simulink model "gm_sampleModel1687_3_sub"  (R2023a)
settings: Solver=VariableStepAuto  StartTime=0.0  StopTime=10.0  RelTol=1e-3
libraries: hdlsllib x3, simulink x2
settings Model: Creator=user1  LastModifiedBy=user1
settings OptimizationCC: BlockReduction=off  ConditionallyExecuteInputs=off
settings DebuggingCC: InheritedTsInSrcMsg=none

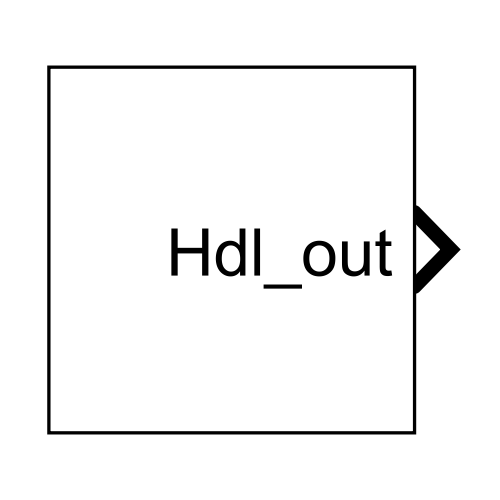
[thumbnail: Simulink's stored preview of the top-level diagram]
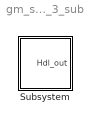
== system gm_sampleModel1687_3_sub ==
  Subsystem : Subsystem

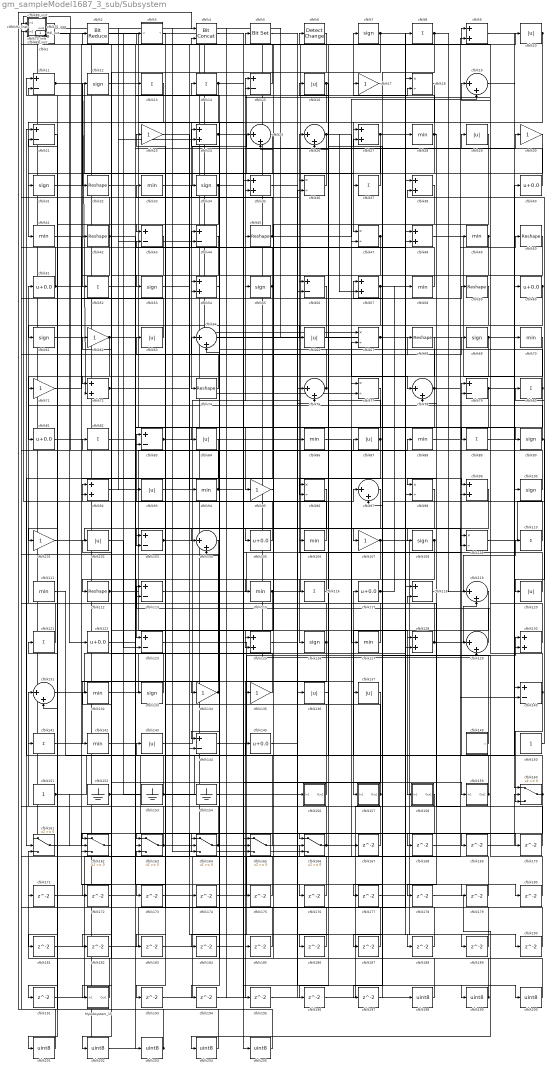
== system gm_sampleModel1687_3_sub/Subsystem ==
  Mysubsystem_15 : Subsystem
  cfblk1 : hdlsllib/Logic and Bit Operations/Bit Slice  lidx=7  ridx=0
  cfblk{10,16,29,63,66,84,87,93,102,120,136..137,143} (13 alike) : Abs  OutDataTypeStr=uint8  SaturateOnIntegerOverflow=off
  cfblk{7,12,31,34,53,55,61,69,90,100,108,126,133} (13 alike) : Signum
  cfblk{17,23,30,62,71,95,101,107,134..135} (10 alike) : Gain  OutDataTypeStr=uint8
  cfblk{11,15,21,43..44,56,79,83,103,113,118,123,140,144} (14 alike) : Sum  Inputs=+-  OutDataTypeStr=uint8
  cfblk{19,25..26,64,76,78,97,104,119,129,131} (11 alike) : Sum  Inputs=|++  OutDataTypeStr=uint8
  cfblk{40,51,60,81,105,117,122,145} (8 alike) : Bias  Bias=0.0  SaturateOnIntegerOverflow=off
  cfblk{28,33,41,49,58,70,86,88,94,106,111,115,127,132,142} (15 alike) : MinMax  OutDataTypeStr=uint8
  cfblk{18,36,47,67,77,96,98,109} (8 alike) : Product  Inputs=*/  OutDataTypeStr=uint8  RndMeth=Zero  SaturateOnIntegerOverflow=on
  cfblk{8,13..14,37,52,80,82,89,110,116,121,141} (12 alike) : Sum  Inputs=+  OutDataTypeStr=uint8
  cfblk{32,42,45,50,59,68,74,112} (8 alike) : Reshape
  cfblk114_inst : Subsystem
  cfblk124_inst : Subsystem
  cfblk{9,24,27,35,38,48,54,57,72,92,99,125,128,130} (14 alike) : Sum  OutDataTypeStr=uint8
  cfblk138_inst : Subsystem
  cfblk149 : Subsystem  mask(Counter Limited){uplimit=double(7), tsamp=double(-1)}
      mask prompts: uplimit "Simulink:masks:UpperLimit_MP"; tsamp "Simulink:masks:SampleTime_MP"
      mask help: Simulink:masks:CounterLimited_MD
      mask init:
      | nbits = double(8);
      | tsamp = double(-1);
      | uplimit = double(7);
  cfblk150 : Constant  OutDataTypeStr=uint8  SampleTime=-1
  cfblk151 : Constant  OutDataTypeStr=uint8  SampleTime=-1
  cfblk152 : Ground
  cfblk153 : Ground
  cfblk154 : Ground
  cfblk156 : Subsystem
  cfblk157 : Subsystem
  cfblk158 : Subsystem
  cfblk159 : Subsystem
  cfblk{160..166} (7 alike) : Switch  OutDataTypeStr=uint8  SaturateOnIntegerOverflow=off  InputSameDT=off
  cfblk{167..191,193..197} (30 alike) : Delay  SampleTime=1
  cfblk{198..205} (8 alike) : DataTypeConversion  OutDataTypeStr=uint8  SaturateOnIntegerOverflow=off  RndMeth=Floor
  cfblk2 : hdlsllib/Logic and Bit Operations/Bit Reduce  mode=AND
  cfblk20_inst : Subsystem
  cfblk22_inst : Subsystem
  cfblk3 : Subsystem  mask(Detect Rise Positive){vinit=double(0), InputProcessing=Elements as channels (sample based), OutDataTypeStr=uint8}
      mask prompts: vinit "Simulink:masks:InitialCondition_MP"; InputProcessing "Simulink:masks:InputProcessing_MP"; OutDataTypeStr "Simulink:masks:OutputDataType_MP"
      mask help: Simulink:masks:DetectRisePositive_MD
      mask init:
      | InputProcessing = 'Elements as channels (sample based)';
      | OutDataTypeStr = 'uint8';
      | vinit = double(0);
      mask TypeOptions InputProcessing: Simulink:masks:ColumnsAsChannelsFrameBased | Simulink:masks:ElementsAsChannelsSampleBased
      mask TypeOptions OutDataTypeStr: Simulink:masks:uint8 | Simulink:masks:boolean
      mask Display: fprintf('U > 0\n&  NOT\nU/z > 0')
  cfblk39_inst : Subsystem
  cfblk4 : hdlsllib/Logic and Bit Operations/Bit Concat  numInputs=2
  cfblk46_inst : Subsystem
  cfblk5 : simulink/Logic and Bit Operations/Bit Set  iBit=0
      settings: LibrarySourceBlock=|
      | hdlsllib/Logic and Bit
      | Operations/Bit Set
  cfblk6 : simulink/Logic and Bit Operations/Detect Change  vinit=0  OutDataTypeStr=uint8
      settings: LibrarySourceBlock=|
      | hdlsllib/Logic and Bit
      | Operations/Detect
      | Change
  cfblk65_inst : Subsystem
  cfblk73_inst : Subsystem
  cfblk75_inst : Subsystem
  cfblk85_inst : Subsystem
  cfblk91_inst : Subsystem
  Hdl_out : Outport  OutDataTypeStr=uint8  SampleTime=1
  wires:
  Mysubsystem_15/1(Out1) -> cfblk161/3
  cfblk1/1 -> cfblk122/1
  cfblk10/1 -> cfblk74/1, cfblk47/1
  cfblk100/1 -> cfblk65_inst/1(in1)
  cfblk101/1 -> cfblk105/1
  cfblk102/1 -> cfblk123/2
  cfblk103/1 -> cfblk15/1, cfblk173/1
  cfblk104/1 -> cfblk142/1
  cfblk105/1 -> cfblk83/1
  cfblk106/1 -> cfblk75_inst/2(in2)
  cfblk107/1 -> cfblk123/1, cfblk189/1
  cfblk108/1 -> cfblk126/1, cfblk112/1
  cfblk109/1 -> cfblk38/2
  cfblk11/1 -> cfblk72/2, cfblk37/1
  cfblk110/1 -> cfblk45/1
  cfblk111/1 -> cfblk143/1
  cfblk112/1 -> cfblk158/1(In1), cfblk88/1
  cfblk113/1 -> cfblk79/1
  cfblk114_inst/1(out1) -> cfblk70/1
  cfblk115/1 -> cfblk9/1, cfblk162/1
  cfblk116/1 -> cfblk26/1
  cfblk117/1 -> cfblk97/2, cfblk58/1
  cfblk118/1 -> cfblk110/1
  cfblk119/1 -> cfblk157/1(In1)
  cfblk12/1 -> cfblk136/1
  cfblk120/1 -> cfblk56/1
  cfblk121/1 -> cfblk51/1
  cfblk122/1 -> cfblk36/1
  cfblk123/1 -> cfblk188/1
  cfblk124_inst/1(out1) -> cfblk203/1
  cfblk125/1 -> cfblk170/1
  cfblk126/1 -> cfblk24/1, cfblk195/1
  cfblk127/1 -> cfblk16/1
  cfblk128/1 -> cfblk20_inst/1(in1), cfblk119/2, cfblk82/1
  cfblk129/1 -> cfblk35/2
  cfblk13/1 -> cfblk52/1
  cfblk130/1 -> cfblk15/2
  cfblk131/1 -> cfblk48/2
  cfblk132/1 -> cfblk8/1
  cfblk133/1 -> cfblk102/1
  cfblk134/1 -> cfblk46_inst/2(in2), cfblk33/1
  cfblk135/1 -> cfblk62/1
  cfblk136/1 -> cfblk106/1
  cfblk137/1 -> cfblk202/1
  cfblk138_inst/1(out1) -> cfblk86/1
  cfblk14/1 -> cfblk159/1(In1), cfblk41/1
  cfblk140/1 -> cfblk91_inst/2(in2), cfblk160/3, cfblk113/1
  cfblk141/1 -> cfblk168/1
  cfblk142/1 -> cfblk97/1
  cfblk143/1 -> cfblk28/1
  cfblk144/1 -> cfblk130/1
  cfblk145/1 -> cfblk76/1
  cfblk149/1(y) -> cfblk57/1
  cfblk15/1 -> cfblk114_inst/2(in2)
  cfblk150/1 -> cfblk80/1
  cfblk151/1 -> cfblk76/2, cfblk40/1, cfblk162/2
  cfblk152/1 -> cfblk164/3, cfblk117/1, cfblk132/1
  cfblk153/1 -> cfblk56/2, cfblk21/2
  cfblk154/1 -> cfblk1/1
  cfblk156/1(Out1) -> cfblk23/1
  cfblk157/1(Out1) -> cfblk44/1, cfblk145/1
  cfblk158/1(Out1) -> cfblk165/2
  cfblk159/1(Out1) -> cfblk79/2, cfblk6/1
  cfblk16/1 -> cfblk144/1, cfblk186/1
  cfblk160/1 -> cfblk21/1, cfblk193/1
  cfblk161/1 -> cfblk164/1
  cfblk162/1 -> cfblk92/1
  cfblk163/1 -> cfblk22_inst/2(in2), cfblk169/1
  cfblk164/1 -> cfblk131/1, cfblk121/1
  cfblk165/1 -> cfblk93/1
  cfblk166/1 -> cfblk73_inst/1(in1), cfblk196/1
  cfblk167/1 -> cfblk75_inst/1(in1)
  cfblk168/1 -> cfblk140/2
  cfblk169/1 -> cfblk160/2
  cfblk17/1 -> cfblk107/1
  cfblk170/1 -> cfblk118/2
  cfblk171/1 -> cfblk164/2
  cfblk172/1 -> cfblk48/1
  cfblk173/1 -> cfblk99/2
  cfblk174/1 -> cfblk18/1
  cfblk175/1 -> cfblk43/2
  cfblk176/1 -> cfblk91_inst/1(in1)
  cfblk177/1 -> cfblk38/1
  cfblk178/1 -> cfblk204/1
  cfblk179/1 -> cfblk64/2
  cfblk18/1 -> cfblk42/1
  cfblk180/1 -> cfblk129/1
  cfblk181/1 -> cfblk77/1
  cfblk182/1 -> cfblk128/2
  cfblk183/1 -> cfblk166/2
  cfblk184/1 -> cfblk35/1
  cfblk185/1 -> cfblk73_inst/2(in2)
  cfblk186/1 -> cfblk22_inst/1(in1)
  cfblk187/1 -> cfblk65_inst/2(in2)
  cfblk188/1 -> cfblk39_inst/1(in1)
  cfblk189/1 -> cfblk163/3
  cfblk19/1 -> cfblk160/1
  cfblk190/1 -> cfblk131/2
  cfblk191/1 -> cfblk165/1
  cfblk193/1 -> cfblk67/2
  cfblk194/1 -> cfblk109/1
  cfblk195/1 -> cfblk36/2
  cfblk196/1 -> cfblk9/2
  cfblk197/1 -> cfblk27/2
  cfblk198/1 -> cfblk5/1
  cfblk199/1 -> cfblk104/2, cfblk171/1
  cfblk2/1 -> cfblk205/1
  cfblk20_inst/1(out1) -> cfblk161/1, cfblk133/1
  cfblk200/1 -> cfblk2/1
  cfblk201/1 -> cfblk4/1
  cfblk202/1 -> cfblk4/2
  cfblk203/1 -> cfblk85_inst/2(in2), cfblk141/1
  cfblk204/1 -> cfblk124_inst/1(in1)
  cfblk205/1 -> cfblk124_inst/2(in2)
  cfblk21/1 -> cfblk201/1
  cfblk22_inst/1(out1) -> cfblk24/2, cfblk198/1
  cfblk23/1 -> cfblk108/1
  cfblk24/1 -> cfblk47/2, cfblk134/1
  cfblk25/1 -> cfblk163/1
  cfblk26/1 -> cfblk78/1, cfblk57/2, cfblk54/2
  cfblk27/1 -> cfblk101/1, cfblk89/1
  cfblk28/1 -> cfblk7/1, cfblk144/2, cfblk98/1, cfblk191/1
  cfblk29/1 -> cfblk187/1
  cfblk3/1(Y) -> cfblk53/1
  cfblk30/1 -> cfblk182/1
  cfblk31/1 -> cfblk12/1
  cfblk32/1 -> cfblk17/1
  cfblk33/1 -> cfblk18/2
  cfblk34/1 -> cfblk30/1, cfblk183/1, cfblk181/1
  cfblk35/1 -> cfblk128/1
  cfblk36/1 -> cfblk31/1
  cfblk37/1 -> cfblk138_inst/1(in1)
  cfblk38/1 -> cfblk115/1
  cfblk39_inst/1(out1) -> cfblk67/1
  cfblk4/1 -> cfblk200/1
  cfblk40/1 -> cfblk25/1
  cfblk41/1 -> cfblk179/1
  cfblk42/1 -> cfblk90/1, cfblk162/3, cfblk11/2
  cfblk43/1 -> cfblk72/1
  cfblk44/1 -> cfblk54/1
  cfblk45/1 -> cfblk85_inst/1(in1), cfblk19/2
  cfblk46_inst/1(out1) -> cfblk111/1, cfblk13/1
  cfblk47/1 -> cfblk84/1, cfblk96/2
  cfblk48/1 -> cfblk100/1
  cfblk49/1 -> cfblk165/3, cfblk194/1
  cfblk5/1 -> cfblk199/1
  cfblk50/1 -> cfblk83/2
  cfblk51/1 -> cfblk163/2, cfblk137/1, cfblk114_inst/1(in1)
  cfblk52/1 -> cfblk29/1
  cfblk53/1 -> cfblk99/1
  cfblk54/1 -> cfblk14/1
  cfblk55/1 -> cfblk161/2, cfblk138_inst/2(in2)
  cfblk56/1 -> cfblk66/1
  cfblk57/1 -> cfblk125/2, cfblk180/1
  cfblk58/1 -> cfblk26/2
  cfblk59/1 -> cfblk116/1
  cfblk6/1 -> cfblk43/1
  cfblk60/1 -> cfblk104/1, cfblk197/1
  cfblk61/1 -> cfblk3/1(U)
  cfblk62/1 -> cfblk92/2, cfblk175/1, cfblk174/1
  cfblk63/1 -> cfblk46_inst/1(in1)
  cfblk64/1 -> cfblk109/2
  cfblk65_inst/1(out1) -> cfblk44/2, cfblk166/3, cfblk167/1
  cfblk66/1 -> cfblk61/1
  cfblk67/1 -> cfblk118/1, Hdl_out/1
  cfblk68/1 -> cfblk81/1
  cfblk69/1 -> cfblk78/2, cfblk19/1
  cfblk7/1 -> cfblk32/1, cfblk190/1
  cfblk70/1 -> cfblk172/1
  cfblk71/1 -> cfblk59/1
  cfblk72/1 -> cfblk98/2, cfblk135/1
  cfblk73_inst/1(out1) -> cfblk156/1(In1)
  cfblk74/1 -> cfblk39_inst/2(in2)
  cfblk75_inst/1(out1) -> cfblk94/1
  cfblk76/1 -> cfblk63/1, cfblk55/1
  cfblk77/1 -> cfblk95/1
  cfblk78/1 -> cfblk50/1, cfblk34/1, cfblk113/2
  cfblk79/1 -> cfblk130/2, cfblk178/1
  cfblk8/1 -> cfblk27/1, cfblk119/1
  cfblk80/1 -> cfblk11/1, cfblk103/2
  cfblk81/1 -> cfblk96/1
  cfblk82/1 -> cfblk69/1
  cfblk83/1 -> cfblk68/1, cfblk185/1
  cfblk84/1 -> Mysubsystem_15/1(In1)
  cfblk85_inst/1(out1) -> cfblk77/2
  cfblk86/1 -> cfblk127/1
  cfblk87/1 -> cfblk64/1, cfblk166/1
  cfblk88/1 -> cfblk49/1
  cfblk89/1 -> cfblk60/1
  cfblk9/1 -> cfblk140/1
  cfblk90/1 -> cfblk120/1, cfblk71/1
  cfblk91_inst/1(out1) -> cfblk129/2
  cfblk92/1 -> cfblk176/1
  cfblk93/1 -> cfblk10/1
  cfblk94/1 -> cfblk87/1, cfblk20_inst/2(in2)
  cfblk95/1 -> cfblk25/2
  cfblk96/1 -> cfblk184/1
  cfblk97/1 -> cfblk125/1
  cfblk98/1 -> cfblk177/1
  cfblk99/1 -> cfblk103/1

== system gm_sampleModel1687_3_sub/Subsystem/Mysubsystem_15 ==
  In1 : Inport  OutDataTypeStr=uint8  PortDimensions=1  SampleTime=1
  cfblk192 : Delay  SampleTime=1
  Out1 : Outport  SampleTime=1
  wires:
  In1/1 -> cfblk192/1
  cfblk192/1 -> Out1/1

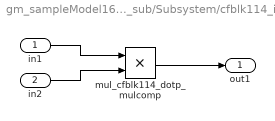
== system gm_sampleModel1687_3_sub/Subsystem/cfblk114_inst ==
  in1 : Inport  OutDataTypeStr=uint8  SampleTime=1
  in2 : Inport  Port=2  OutDataTypeStr=uint8  SampleTime=1
  mul_cfblk114_dotp_mulcomp : Product  Inputs=**  OutDataTypeStr=uint8  SampleTime=1
  out1 : Outport  OutDataTypeStr=uint8  SampleTime=1
  wires:
  in1/1 -> mul_cfblk114_dotp_mulcomp/1
  in2/1 -> mul_cfblk114_dotp_mulcomp/2
  mul_cfblk114_dotp_mulcomp/1 -> out1/1

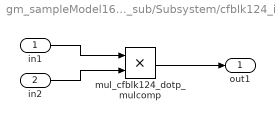
== system gm_sampleModel1687_3_sub/Subsystem/cfblk124_inst ==
  in1 : Inport  OutDataTypeStr=uint8  SampleTime=1
  in2 : Inport  Port=2  OutDataTypeStr=uint8  SampleTime=1
  mul_cfblk124_dotp_mulcomp : Product  Inputs=**  OutDataTypeStr=uint8  SampleTime=1
  out1 : Outport  OutDataTypeStr=uint8  SampleTime=1
  wires:
  in1/1 -> mul_cfblk124_dotp_mulcomp/1
  in2/1 -> mul_cfblk124_dotp_mulcomp/2
  mul_cfblk124_dotp_mulcomp/1 -> out1/1

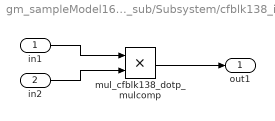
== system gm_sampleModel1687_3_sub/Subsystem/cfblk138_inst ==
  in1 : Inport  OutDataTypeStr=uint8  SampleTime=1
  in2 : Inport  Port=2  OutDataTypeStr=uint8  SampleTime=1
  mul_cfblk138_dotp_mulcomp : Product  Inputs=**  OutDataTypeStr=uint8  SampleTime=1
  out1 : Outport  OutDataTypeStr=uint8  SampleTime=1
  wires:
  in1/1 -> mul_cfblk138_dotp_mulcomp/1
  in2/1 -> mul_cfblk138_dotp_mulcomp/2
  mul_cfblk138_dotp_mulcomp/1 -> out1/1

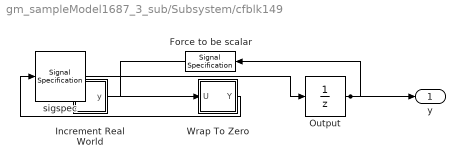
== system gm_sampleModel1687_3_sub/Subsystem/cfblk149 ==
  Force to be scalar : SignalSpecification  DisableCoverage=on  Dimensions=1
  Increment Real World : Subsystem  mask(Real World Value Increment){}
      mask help: Simulink:masks:RealWorldValueIncrement_MD
      mask Display: disp('V++')
  Output : UnitDelay  InitialCondition=0.0  SampleTime=tsamp  HasFrameUpgradeWarning=on
  Wrap To Zero : Subsystem  mask(Wrap To Zero){Threshold=double(7)}
      mask prompts: Threshold "Simulink:masks:Threshold_MP"
      mask help: Simulink:masks:WrapToZero_MD
  sigspec : SignalSpecification  OutDataTypeStr=uint8  Dimensions=1
  y : Outport  SampleTime=1
  wires:
  Force to be scalar/1 -> Increment Real World/1(u)
  Increment Real World/1(y) -> Wrap To Zero/1(U)
  Output/1 -> Force to be scalar/1, y/1
  Wrap To Zero/1(Y) -> sigspec/1
  sigspec/1 -> Output/1

== system gm_sampleModel1687_3_sub/Subsystem/cfblk156 ==
  In1 : Inport  OutDataTypeStr=uint8  PortDimensions=1  SampleTime=1
  Out1 : Outport  SampleTime=1
  wires:
  In1/1 -> Out1/1

== system gm_sampleModel1687_3_sub/Subsystem/cfblk157 ==
  In1 : Inport  OutDataTypeStr=uint8  PortDimensions=1  SampleTime=1
  Out1 : Outport  SampleTime=1
  wires:
  In1/1 -> Out1/1

== system gm_sampleModel1687_3_sub/Subsystem/cfblk158 ==
  In1 : Inport  OutDataTypeStr=uint8  PortDimensions=1  SampleTime=1
  Out1 : Outport  SampleTime=1
  wires:
  In1/1 -> Out1/1

== system gm_sampleModel1687_3_sub/Subsystem/cfblk159 ==
  In1 : Inport  OutDataTypeStr=uint8  PortDimensions=1  SampleTime=1
  Out1 : Outport  SampleTime=1
  wires:
  In1/1 -> Out1/1

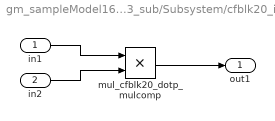
== system gm_sampleModel1687_3_sub/Subsystem/cfblk20_inst ==
  in1 : Inport  OutDataTypeStr=uint8  SampleTime=1
  in2 : Inport  Port=2  OutDataTypeStr=uint8  SampleTime=1
  mul_cfblk20_dotp_mulcomp : Product  Inputs=**  OutDataTypeStr=uint8  SampleTime=1
  out1 : Outport  OutDataTypeStr=uint8  SampleTime=1
  wires:
  in1/1 -> mul_cfblk20_dotp_mulcomp/1
  in2/1 -> mul_cfblk20_dotp_mulcomp/2
  mul_cfblk20_dotp_mulcomp/1 -> out1/1

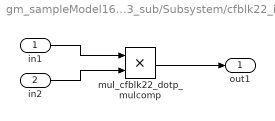
== system gm_sampleModel1687_3_sub/Subsystem/cfblk22_inst ==
  in1 : Inport  OutDataTypeStr=uint8  SampleTime=1
  in2 : Inport  Port=2  OutDataTypeStr=uint8  SampleTime=1
  mul_cfblk22_dotp_mulcomp : Product  Inputs=**  OutDataTypeStr=uint8  SampleTime=1
  out1 : Outport  OutDataTypeStr=uint8  SampleTime=1
  wires:
  in1/1 -> mul_cfblk22_dotp_mulcomp/1
  in2/1 -> mul_cfblk22_dotp_mulcomp/2
  mul_cfblk22_dotp_mulcomp/1 -> out1/1

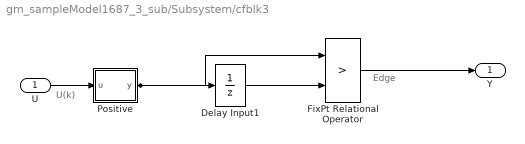
== system gm_sampleModel1687_3_sub/Subsystem/cfblk3 ==
  note: U(k)
  note: Edge
  U : Inport  OutDataTypeStr=uint8  SampleTime=1
  Delay Input1 : UnitDelay  Description=Store in Global RAM  DisableCoverage=on  InitialCondition=vinit  SampleTime=-1  HasFrameUpgradeWarning=on
  FixPt Relational Operator : RelationalOperator  Operator=>  OutDataTypeStr=fixdt(0, 8)  ZeroCross=off  InputSameDT=off
  Positive : Subsystem  mask(Compare To Zero){relop=>, OutDataTypeStr=boolean, ZeroCross=off}
      mask prompts: relop "Simulink:masks:Operator_MP"; OutDataTypeStr "Simulink:masks:OutputDataType_MP"; ZeroCross "Simulink:masks:EnableZerocrossingDetection_MP"
      mask help: Simulink:masks:CompareToZero_MD
      mask init:
      | OutDataTypeStr = 'boolean';
      | ZeroCross = 'off';
      | blkName = 'sampleModel1687_3_sub/Subsystem/cfblk3/Positive';
      | relop = '>';
      | setValue = 'boolean';
      mask TypeOptions relop: == | ~= | < | <= | >= | >
      mask TypeOptions OutDataTypeStr: Simulink:masks:uint8 | Simulink:masks:boolean
      mask Callback ZeroCross: sl('zeroCrossEnable', gcbh);
      mask Display: disp([relop,' 0'])
  Y : Outport  SampleTime=1
  wires:
  U/1 -> Positive/1(u)
  Delay Input1/1 -> FixPt Relational Operator/2
  FixPt Relational Operator/1 -> Y/1
  Positive/1(y) -> FixPt Relational Operator/1, Delay Input1/1

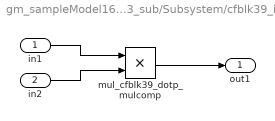
== system gm_sampleModel1687_3_sub/Subsystem/cfblk39_inst ==
  in1 : Inport  OutDataTypeStr=uint8  SampleTime=1
  in2 : Inport  Port=2  OutDataTypeStr=uint8  SampleTime=1
  mul_cfblk39_dotp_mulcomp : Product  Inputs=**  OutDataTypeStr=uint8  SampleTime=1
  out1 : Outport  OutDataTypeStr=uint8  SampleTime=1
  wires:
  in1/1 -> mul_cfblk39_dotp_mulcomp/1
  in2/1 -> mul_cfblk39_dotp_mulcomp/2
  mul_cfblk39_dotp_mulcomp/1 -> out1/1

== system gm_sampleModel1687_3_sub/Subsystem/cfblk46_inst ==
  in1 : Inport  OutDataTypeStr=uint8  SampleTime=1
  in2 : Inport  Port=2  OutDataTypeStr=uint8  SampleTime=1
  mul_cfblk46_dotp_mulcomp : Product  Inputs=**  OutDataTypeStr=uint8  SampleTime=1
  out1 : Outport  OutDataTypeStr=uint8  SampleTime=1
  wires:
  in1/1 -> mul_cfblk46_dotp_mulcomp/1
  in2/1 -> mul_cfblk46_dotp_mulcomp/2
  mul_cfblk46_dotp_mulcomp/1 -> out1/1

== system gm_sampleModel1687_3_sub/Subsystem/cfblk65_inst ==
  in1 : Inport  OutDataTypeStr=uint8  SampleTime=1
  in2 : Inport  Port=2  OutDataTypeStr=uint8  SampleTime=1
  mul_cfblk65_dotp_mulcomp : Product  Inputs=**  OutDataTypeStr=uint8  SampleTime=1
  out1 : Outport  OutDataTypeStr=uint8  SampleTime=1
  wires:
  in1/1 -> mul_cfblk65_dotp_mulcomp/1
  in2/1 -> mul_cfblk65_dotp_mulcomp/2
  mul_cfblk65_dotp_mulcomp/1 -> out1/1

== system gm_sampleModel1687_3_sub/Subsystem/cfblk73_inst ==
  in1 : Inport  OutDataTypeStr=uint8  SampleTime=1
  in2 : Inport  Port=2  OutDataTypeStr=uint8  SampleTime=1
  mul_cfblk73_dotp_mulcomp : Product  Inputs=**  OutDataTypeStr=uint8  SampleTime=1
  out1 : Outport  OutDataTypeStr=uint8  SampleTime=1
  wires:
  in1/1 -> mul_cfblk73_dotp_mulcomp/1
  in2/1 -> mul_cfblk73_dotp_mulcomp/2
  mul_cfblk73_dotp_mulcomp/1 -> out1/1

== system gm_sampleModel1687_3_sub/Subsystem/cfblk75_inst ==
  in1 : Inport  OutDataTypeStr=uint8  SampleTime=1
  in2 : Inport  Port=2  OutDataTypeStr=uint8  SampleTime=1
  mul_cfblk75_dotp_mulcomp : Product  Inputs=**  OutDataTypeStr=uint8  SampleTime=1
  out1 : Outport  OutDataTypeStr=uint8  SampleTime=1
  wires:
  in1/1 -> mul_cfblk75_dotp_mulcomp/1
  in2/1 -> mul_cfblk75_dotp_mulcomp/2
  mul_cfblk75_dotp_mulcomp/1 -> out1/1

== system gm_sampleModel1687_3_sub/Subsystem/cfblk85_inst ==
  in1 : Inport  OutDataTypeStr=uint8  SampleTime=1
  in2 : Inport  Port=2  OutDataTypeStr=uint8  SampleTime=1
  mul_cfblk85_dotp_mulcomp : Product  Inputs=**  OutDataTypeStr=uint8  SampleTime=1
  out1 : Outport  OutDataTypeStr=uint8  SampleTime=1
  wires:
  in1/1 -> mul_cfblk85_dotp_mulcomp/1
  in2/1 -> mul_cfblk85_dotp_mulcomp/2
  mul_cfblk85_dotp_mulcomp/1 -> out1/1

== system gm_sampleModel1687_3_sub/Subsystem/cfblk91_inst ==
  in1 : Inport  OutDataTypeStr=uint8  SampleTime=1
  in2 : Inport  Port=2  OutDataTypeStr=uint8  SampleTime=1
  mul_cfblk91_dotp_mulcomp : Product  Inputs=**  OutDataTypeStr=uint8  SampleTime=1
  out1 : Outport  OutDataTypeStr=uint8  SampleTime=1
  wires:
  in1/1 -> mul_cfblk91_dotp_mulcomp/1
  in2/1 -> mul_cfblk91_dotp_mulcomp/2
  mul_cfblk91_dotp_mulcomp/1 -> out1/1

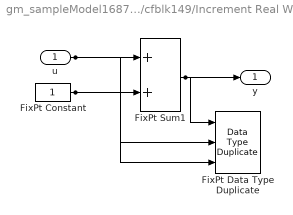
== system gm_sampleModel1687_3_sub/Subsystem/cfblk149/Increment Real World ==
  u : Inport  OutDataTypeStr=uint8  SampleTime=1
  FixPt Constant : Constant  DisableCoverage=on  OutDataTypeStr=Inherit: Inherit via back propagation  SampleTime=-1
  FixPt Data Type Duplicate : DataTypeDuplicate  DisableCoverage=on  NumInputPorts=3
  FixPt Sum1 : Sum  InputSameDT=on  OutDataTypeStr=Inherit: Inherit via back propagation  LockScale=on
  y : Outport  SampleTime=1
  wires:
  u/1 -> FixPt Sum1/1, FixPt Data Type Duplicate/2
  FixPt Constant/1 -> FixPt Sum1/2, FixPt Data Type Duplicate/3
  FixPt Sum1/1 -> FixPt Data Type Duplicate/1, y/1

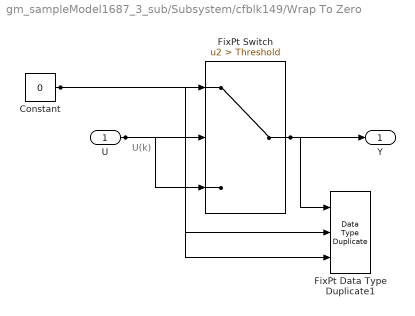
== system gm_sampleModel1687_3_sub/Subsystem/cfblk149/Wrap To Zero ==
  note: U(k)
  U : Inport  OutDataTypeStr=uint8  SampleTime=1
  Constant : Constant  DisableCoverage=on  Value=0  OutDataTypeStr=Inherit: Inherit via back propagation  SampleTime=-1
  FixPt Data Type Duplicate1 : DataTypeDuplicate  DisableCoverage=on  NumInputPorts=3
  FixPt Switch : Switch  Criteria=u2 > Threshold  Threshold=Threshold  OutDataTypeStr=Inherit: Inherit via back propagation  ZeroCross=off  SaturateOnIntegerOverflow=off  InputSameDT=off
  Y : Outport  SampleTime=1
  wires:
  U/1 -> FixPt Switch/3, FixPt Switch/2, FixPt Data Type Duplicate1/2
  Constant/1 -> FixPt Switch/1, FixPt Data Type Duplicate1/3
  FixPt Switch/1 -> FixPt Data Type Duplicate1/1, Y/1

== system gm_sampleModel1687_3_sub/Subsystem/cfblk3/Positive ==
  u : Inport  OutDataTypeStr=uint8  SampleTime=1
  Compare : RelationalOperator  Operator=>  OutDataTypeStr=boolean  ZeroCross=off
  Constant : Constant  DisableCoverage=on  Value=0  OutDataTypeStr=Inherit: Inherit via back propagation  SampleTime=-1  PreserveConstantTs=on
  y : Outport  SampleTime=1
  wires:
  u/1 -> Compare/1
  Compare/1 -> y/1
  Constant/1 -> Compare/2
